simulink model "waterTank3"  (R2015a)
settings: Solver=ode1  StartTime=0.0  StopTime=60  FixedStep=0.5  RelTol=1e-3
values from neighbouring files (symbols this model uses):
  h_0 = .13    (= 0.13)    [script.m]
  k = (r*r*sqrt(2*g))/(R*R)    [script.m]
settings Model: Creator=student  LastModifiedBy=student

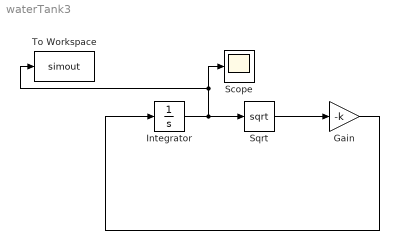
== system waterTank3 ==
  Gain : Gain  Gain=-k
  Integrator : Integrator  InitialCondition=h_0
  Scope : Scope
  Sqrt : Sqrt  SaturateOnIntegerOverflow=on
  To Workspace : ToWorkspace  VariableName=simout  SaveFormat=Timeseries  SampleTime=-1
  wires:
  Integrator/1 -> Scope/1, To Workspace/1, Sqrt/1
  Sqrt/1 -> Gain/1
  Gain/1 -> Integrator/1
